simulink model "p8"  (R2018a)
settings: Solver=VariableStepAuto  StartTime=0.0  StopTime=10.0  RelTol=1e-3
settings Model: Creator=Hassan  LastModifiedBy=Hassan

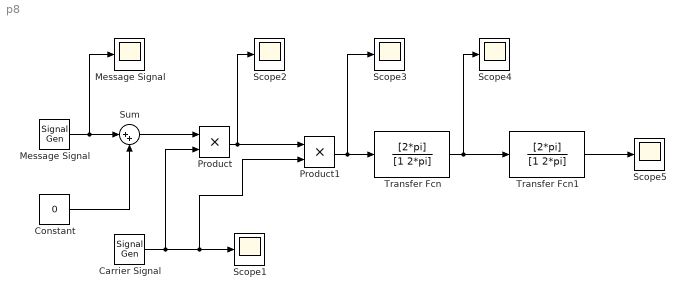
== system p8 ==
  "Carrier Signal " : SignalGenerator  Amplitude=2  Frequency=50  Units=rad/sec
  Constant : Constant  Value=0
  Message Signal : Scope
  "Message Signal " : SignalGenerator  Frequency=5  Units=rad/sec
  Product : Product
  Product1 : Product
  Scope{1..5} (5 alike) : Scope
  Sum : Sum  Inputs=|++
  Transfer Fcn : TransferFcn  Numerator=[2*pi]  Denominator=[1 2*pi]
  Transfer Fcn1 : TransferFcn  Numerator=[2*pi]  Denominator=[1 2*pi]
  wires:
  "Message Signal "/1 -> Message Signal/1, Sum/1
  Sum/1 -> Product/1
  "Carrier Signal "/1 -> Product/2, Product1/2, Scope1/1
  Product/1 -> Scope2/1, Product1/1
  Product1/1 -> Scope3/1, Transfer Fcn/1
  Transfer Fcn/1 -> Transfer Fcn1/1, Scope4/1
  Constant/1 -> Sum/2
  Transfer Fcn1/1 -> Scope5/1
